simulink model "sim_model"  (R2015b)
settings: Solver=FixedStepDiscrete  SolverMode=SingleTasking  StartTime=0.0  StopTime=sim_len  FixedStep=1  RelTol=1e-3
undefined symbols (not defined in the file): A, B, C, ir_matrix, modulator_reg_1_address, modulator_reg_1_default, modulator_reg_1_num_bits, N_sub
libraries: xbsIndex_r4 x3875
(part 4 of 193)

== system sim_model/channelizer/poly_phase_filter1/filter_pipeline_89_taps3/8_taps ==
  delay_line_in : Inport
  result_in : Inport  Port=2
  reset_in : Inport  Port=3
  enable_in : Inport  Port=4
  one_tab_1 : Subsystem  mask{impulse_response_matrix=impulse_response_matrix(2,:), N_sub=N_sub}
      mask prompts: impulse_response_matrix "Tab IR"
  one_tab_2 : Subsystem  mask{impulse_response_matrix=impulse_response_matrix(4,:), N_sub=N_sub}
      mask prompts: impulse_response_matrix "Tab IR"
  one_tab_3 : Subsystem  mask{impulse_response_matrix=impulse_response_matrix(3,:), N_sub=N_sub}
      mask prompts: impulse_response_matrix "Tab IR"
  one_tab_4 : Subsystem  mask{impulse_response_matrix=impulse_response_matrix(6,:), N_sub=N_sub}
      mask prompts: impulse_response_matrix "Tab IR"
  one_tab_5 : Subsystem  mask{impulse_response_matrix=impulse_response_matrix(5,:), N_sub=N_sub}
      mask prompts: impulse_response_matrix "Tab IR"
  one_tab_6 : Subsystem  mask{impulse_response_matrix=impulse_response_matrix(8,:), N_sub=N_sub}
      mask prompts: impulse_response_matrix "Tab IR"
  one_tab_7 : Subsystem  mask{impulse_response_matrix=impulse_response_matrix(7,:), N_sub=N_sub}
      mask prompts: impulse_response_matrix "Tab IR"
  one_tab_8 : Subsystem  mask{impulse_response_matrix=impulse_response_matrix(1,:), N_sub=N_sub}
      mask prompts: impulse_response_matrix "Tab IR"
  delay_line_out : Outport
  result_out : Outport  Port=2
  reset_out : Outport  Port=3
  enable_out : Outport  Port=4
  wires:
  one_tab_6/1(delay_line_out) -> delay_line_out/1
  one_tab_6/2(result_out) -> result_out/1
  one_tab_6/3(reset_out) -> reset_out/1
  result_in/1 -> one_tab_8/2(result_in)
  delay_line_in/1 -> one_tab_8/1(delay_line_in)
  reset_in/1 -> one_tab_8/3(reset_in)
  enable_in/1 -> one_tab_8/4(enable_in)
  one_tab_6/4(enable_out) -> enable_out/1
  one_tab_8/1(delay_line_out) -> one_tab_1/1(delay_line_in)
  one_tab_8/2(result_out) -> one_tab_1/2(result_in)
  one_tab_8/3(reset_out) -> one_tab_1/3(reset_in)
  one_tab_8/4(enable_out) -> one_tab_1/4(enable_in)
  one_tab_3/1(delay_line_out) -> one_tab_2/1(delay_line_in)
  one_tab_3/2(result_out) -> one_tab_2/2(result_in)
  one_tab_3/3(reset_out) -> one_tab_2/3(reset_in)
  one_tab_3/4(enable_out) -> one_tab_2/4(enable_in)
  one_tab_1/1(delay_line_out) -> one_tab_3/1(delay_line_in)
  one_tab_1/2(result_out) -> one_tab_3/2(result_in)
  one_tab_1/3(reset_out) -> one_tab_3/3(reset_in)
  one_tab_1/4(enable_out) -> one_tab_3/4(enable_in)
  one_tab_5/1(delay_line_out) -> one_tab_4/1(delay_line_in)
  one_tab_5/2(result_out) -> one_tab_4/2(result_in)
  one_tab_5/3(reset_out) -> one_tab_4/3(reset_in)
  one_tab_5/4(enable_out) -> one_tab_4/4(enable_in)
  one_tab_2/1(delay_line_out) -> one_tab_5/1(delay_line_in)
  one_tab_2/2(result_out) -> one_tab_5/2(result_in)
  one_tab_2/3(reset_out) -> one_tab_5/3(reset_in)
  one_tab_2/4(enable_out) -> one_tab_5/4(enable_in)
  one_tab_7/1(delay_line_out) -> one_tab_6/1(delay_line_in)
  one_tab_7/2(result_out) -> one_tab_6/2(result_in)
  one_tab_7/3(reset_out) -> one_tab_6/3(reset_in)
  one_tab_7/4(enable_out) -> one_tab_6/4(enable_in)
  one_tab_4/1(delay_line_out) -> one_tab_7/1(delay_line_in)
  one_tab_4/2(result_out) -> one_tab_7/2(result_in)
  one_tab_4/3(reset_out) -> one_tab_7/3(reset_in)
  one_tab_4/4(enable_out) -> one_tab_7/4(enable_in)

== system sim_model/channelizer/poly_phase_filter1/filter_pipeline_89_taps3/8_taps1 ==
  delay_line_in : Inport
  result_in : Inport  Port=2
  reset_in : Inport  Port=3
  enable_in : Inport  Port=4
  one_tab_1 : Subsystem  mask{impulse_response_matrix=impulse_response_matrix(2,:), N_sub=N_sub}
      mask prompts: impulse_response_matrix "Tab IR"
  one_tab_2 : Subsystem  mask{impulse_response_matrix=impulse_response_matrix(4,:), N_sub=N_sub}
      mask prompts: impulse_response_matrix "Tab IR"
  one_tab_3 : Subsystem  mask{impulse_response_matrix=impulse_response_matrix(3,:), N_sub=N_sub}
      mask prompts: impulse_response_matrix "Tab IR"
  one_tab_4 : Subsystem  mask{impulse_response_matrix=impulse_response_matrix(6,:), N_sub=N_sub}
      mask prompts: impulse_response_matrix "Tab IR"
  one_tab_5 : Subsystem  mask{impulse_response_matrix=impulse_response_matrix(5,:), N_sub=N_sub}
      mask prompts: impulse_response_matrix "Tab IR"
  one_tab_6 : Subsystem  mask{impulse_response_matrix=impulse_response_matrix(8,:), N_sub=N_sub}
      mask prompts: impulse_response_matrix "Tab IR"
  one_tab_7 : Subsystem  mask{impulse_response_matrix=impulse_response_matrix(7,:), N_sub=N_sub}
      mask prompts: impulse_response_matrix "Tab IR"
  one_tab_8 : Subsystem  mask{impulse_response_matrix=impulse_response_matrix(1,:), N_sub=N_sub}
      mask prompts: impulse_response_matrix "Tab IR"
  delay_line_out : Outport
  result_out : Outport  Port=2
  reset_out : Outport  Port=3
  enable_out : Outport  Port=4
  wires:
  one_tab_6/1(delay_line_out) -> delay_line_out/1
  one_tab_6/2(result_out) -> result_out/1
  one_tab_6/3(reset_out) -> reset_out/1
  result_in/1 -> one_tab_8/2(result_in)
  delay_line_in/1 -> one_tab_8/1(delay_line_in)
  reset_in/1 -> one_tab_8/3(reset_in)
  enable_in/1 -> one_tab_8/4(enable_in)
  one_tab_6/4(enable_out) -> enable_out/1
  one_tab_8/1(delay_line_out) -> one_tab_1/1(delay_line_in)
  one_tab_8/2(result_out) -> one_tab_1/2(result_in)
  one_tab_8/3(reset_out) -> one_tab_1/3(reset_in)
  one_tab_8/4(enable_out) -> one_tab_1/4(enable_in)
  one_tab_3/1(delay_line_out) -> one_tab_2/1(delay_line_in)
  one_tab_3/2(result_out) -> one_tab_2/2(result_in)
  one_tab_3/3(reset_out) -> one_tab_2/3(reset_in)
  one_tab_3/4(enable_out) -> one_tab_2/4(enable_in)
  one_tab_1/1(delay_line_out) -> one_tab_3/1(delay_line_in)
  one_tab_1/2(result_out) -> one_tab_3/2(result_in)
  one_tab_1/3(reset_out) -> one_tab_3/3(reset_in)
  one_tab_1/4(enable_out) -> one_tab_3/4(enable_in)
  one_tab_5/1(delay_line_out) -> one_tab_4/1(delay_line_in)
  one_tab_5/2(result_out) -> one_tab_4/2(result_in)
  one_tab_5/3(reset_out) -> one_tab_4/3(reset_in)
  one_tab_5/4(enable_out) -> one_tab_4/4(enable_in)
  one_tab_2/1(delay_line_out) -> one_tab_5/1(delay_line_in)
  one_tab_2/2(result_out) -> one_tab_5/2(result_in)
  one_tab_2/3(reset_out) -> one_tab_5/3(reset_in)
  one_tab_2/4(enable_out) -> one_tab_5/4(enable_in)
  one_tab_7/1(delay_line_out) -> one_tab_6/1(delay_line_in)
  one_tab_7/2(result_out) -> one_tab_6/2(result_in)
  one_tab_7/3(reset_out) -> one_tab_6/3(reset_in)
  one_tab_7/4(enable_out) -> one_tab_6/4(enable_in)
  one_tab_4/1(delay_line_out) -> one_tab_7/1(delay_line_in)
  one_tab_4/2(result_out) -> one_tab_7/2(result_in)
  one_tab_4/3(reset_out) -> one_tab_7/3(reset_in)
  one_tab_4/4(enable_out) -> one_tab_7/4(enable_in)

== system sim_model/channelizer/poly_phase_filter1/filter_pipeline_89_taps3/8_taps10 ==
  delay_line_in : Inport
  result_in : Inport  Port=2
  reset_in : Inport  Port=3
  enable_in : Inport  Port=4
  one_tab_1 : Subsystem  mask{impulse_response_matrix=impulse_response_matrix(2,:), N_sub=N_sub}
      mask prompts: impulse_response_matrix "Tab IR"
  one_tab_2 : Subsystem  mask{impulse_response_matrix=impulse_response_matrix(4,:), N_sub=N_sub}
      mask prompts: impulse_response_matrix "Tab IR"
  one_tab_3 : Subsystem  mask{impulse_response_matrix=impulse_response_matrix(3,:), N_sub=N_sub}
      mask prompts: impulse_response_matrix "Tab IR"
  one_tab_4 : Subsystem  mask{impulse_response_matrix=impulse_response_matrix(6,:), N_sub=N_sub}
      mask prompts: impulse_response_matrix "Tab IR"
  one_tab_5 : Subsystem  mask{impulse_response_matrix=impulse_response_matrix(5,:), N_sub=N_sub}
      mask prompts: impulse_response_matrix "Tab IR"
  one_tab_6 : Subsystem  mask{impulse_response_matrix=impulse_response_matrix(8,:), N_sub=N_sub}
      mask prompts: impulse_response_matrix "Tab IR"
  one_tab_7 : Subsystem  mask{impulse_response_matrix=impulse_response_matrix(7,:), N_sub=N_sub}
      mask prompts: impulse_response_matrix "Tab IR"
  one_tab_8 : Subsystem  mask{impulse_response_matrix=impulse_response_matrix(1,:), N_sub=N_sub}
      mask prompts: impulse_response_matrix "Tab IR"
  delay_line_out : Outport
  result_out : Outport  Port=2
  reset_out : Outport  Port=3
  enable_out : Outport  Port=4
  wires:
  one_tab_6/1(delay_line_out) -> delay_line_out/1
  one_tab_6/2(result_out) -> result_out/1
  one_tab_6/3(reset_out) -> reset_out/1
  result_in/1 -> one_tab_8/2(result_in)
  delay_line_in/1 -> one_tab_8/1(delay_line_in)
  reset_in/1 -> one_tab_8/3(reset_in)
  enable_in/1 -> one_tab_8/4(enable_in)
  one_tab_6/4(enable_out) -> enable_out/1
  one_tab_8/1(delay_line_out) -> one_tab_1/1(delay_line_in)
  one_tab_8/2(result_out) -> one_tab_1/2(result_in)
  one_tab_8/3(reset_out) -> one_tab_1/3(reset_in)
  one_tab_8/4(enable_out) -> one_tab_1/4(enable_in)
  one_tab_3/1(delay_line_out) -> one_tab_2/1(delay_line_in)
  one_tab_3/2(result_out) -> one_tab_2/2(result_in)
  one_tab_3/3(reset_out) -> one_tab_2/3(reset_in)
  one_tab_3/4(enable_out) -> one_tab_2/4(enable_in)
  one_tab_1/1(delay_line_out) -> one_tab_3/1(delay_line_in)
  one_tab_1/2(result_out) -> one_tab_3/2(result_in)
  one_tab_1/3(reset_out) -> one_tab_3/3(reset_in)
  one_tab_1/4(enable_out) -> one_tab_3/4(enable_in)
  one_tab_5/1(delay_line_out) -> one_tab_4/1(delay_line_in)
  one_tab_5/2(result_out) -> one_tab_4/2(result_in)
  one_tab_5/3(reset_out) -> one_tab_4/3(reset_in)
  one_tab_5/4(enable_out) -> one_tab_4/4(enable_in)
  one_tab_2/1(delay_line_out) -> one_tab_5/1(delay_line_in)
  one_tab_2/2(result_out) -> one_tab_5/2(result_in)
  one_tab_2/3(reset_out) -> one_tab_5/3(reset_in)
  one_tab_2/4(enable_out) -> one_tab_5/4(enable_in)
  one_tab_7/1(delay_line_out) -> one_tab_6/1(delay_line_in)
  one_tab_7/2(result_out) -> one_tab_6/2(result_in)
  one_tab_7/3(reset_out) -> one_tab_6/3(reset_in)
  one_tab_7/4(enable_out) -> one_tab_6/4(enable_in)
  one_tab_4/1(delay_line_out) -> one_tab_7/1(delay_line_in)
  one_tab_4/2(result_out) -> one_tab_7/2(result_in)
  one_tab_4/3(reset_out) -> one_tab_7/3(reset_in)
  one_tab_4/4(enable_out) -> one_tab_7/4(enable_in)

== system sim_model/channelizer/poly_phase_filter1/filter_pipeline_89_taps3/8_taps2 ==
  delay_line_in : Inport
  result_in : Inport  Port=2
  reset_in : Inport  Port=3
  enable_in : Inport  Port=4
  one_tab_1 : Subsystem  mask{impulse_response_matrix=impulse_response_matrix(2,:), N_sub=N_sub}
      mask prompts: impulse_response_matrix "Tab IR"
  one_tab_2 : Subsystem  mask{impulse_response_matrix=impulse_response_matrix(4,:), N_sub=N_sub}
      mask prompts: impulse_response_matrix "Tab IR"
  one_tab_3 : Subsystem  mask{impulse_response_matrix=impulse_response_matrix(3,:), N_sub=N_sub}
      mask prompts: impulse_response_matrix "Tab IR"
  one_tab_4 : Subsystem  mask{impulse_response_matrix=impulse_response_matrix(6,:), N_sub=N_sub}
      mask prompts: impulse_response_matrix "Tab IR"
  one_tab_5 : Subsystem  mask{impulse_response_matrix=impulse_response_matrix(5,:), N_sub=N_sub}
      mask prompts: impulse_response_matrix "Tab IR"
  one_tab_6 : Subsystem  mask{impulse_response_matrix=impulse_response_matrix(8,:), N_sub=N_sub}
      mask prompts: impulse_response_matrix "Tab IR"
  one_tab_7 : Subsystem  mask{impulse_response_matrix=impulse_response_matrix(7,:), N_sub=N_sub}
      mask prompts: impulse_response_matrix "Tab IR"
  one_tab_8 : Subsystem  mask{impulse_response_matrix=impulse_response_matrix(1,:), N_sub=N_sub}
      mask prompts: impulse_response_matrix "Tab IR"
  delay_line_out : Outport
  result_out : Outport  Port=2
  reset_out : Outport  Port=3
  enable_out : Outport  Port=4
  wires:
  one_tab_6/1(delay_line_out) -> delay_line_out/1
  one_tab_6/2(result_out) -> result_out/1
  one_tab_6/3(reset_out) -> reset_out/1
  result_in/1 -> one_tab_8/2(result_in)
  delay_line_in/1 -> one_tab_8/1(delay_line_in)
  reset_in/1 -> one_tab_8/3(reset_in)
  enable_in/1 -> one_tab_8/4(enable_in)
  one_tab_6/4(enable_out) -> enable_out/1
  one_tab_8/1(delay_line_out) -> one_tab_1/1(delay_line_in)
  one_tab_8/2(result_out) -> one_tab_1/2(result_in)
  one_tab_8/3(reset_out) -> one_tab_1/3(reset_in)
  one_tab_8/4(enable_out) -> one_tab_1/4(enable_in)
  one_tab_3/1(delay_line_out) -> one_tab_2/1(delay_line_in)
  one_tab_3/2(result_out) -> one_tab_2/2(result_in)
  one_tab_3/3(reset_out) -> one_tab_2/3(reset_in)
  one_tab_3/4(enable_out) -> one_tab_2/4(enable_in)
  one_tab_1/1(delay_line_out) -> one_tab_3/1(delay_line_in)
  one_tab_1/2(result_out) -> one_tab_3/2(result_in)
  one_tab_1/3(reset_out) -> one_tab_3/3(reset_in)
  one_tab_1/4(enable_out) -> one_tab_3/4(enable_in)
  one_tab_5/1(delay_line_out) -> one_tab_4/1(delay_line_in)
  one_tab_5/2(result_out) -> one_tab_4/2(result_in)
  one_tab_5/3(reset_out) -> one_tab_4/3(reset_in)
  one_tab_5/4(enable_out) -> one_tab_4/4(enable_in)
  one_tab_2/1(delay_line_out) -> one_tab_5/1(delay_line_in)
  one_tab_2/2(result_out) -> one_tab_5/2(result_in)
  one_tab_2/3(reset_out) -> one_tab_5/3(reset_in)
  one_tab_2/4(enable_out) -> one_tab_5/4(enable_in)
  one_tab_7/1(delay_line_out) -> one_tab_6/1(delay_line_in)
  one_tab_7/2(result_out) -> one_tab_6/2(result_in)
  one_tab_7/3(reset_out) -> one_tab_6/3(reset_in)
  one_tab_7/4(enable_out) -> one_tab_6/4(enable_in)
  one_tab_4/1(delay_line_out) -> one_tab_7/1(delay_line_in)
  one_tab_4/2(result_out) -> one_tab_7/2(result_in)
  one_tab_4/3(reset_out) -> one_tab_7/3(reset_in)
  one_tab_4/4(enable_out) -> one_tab_7/4(enable_in)

== system sim_model/channelizer/poly_phase_filter1/filter_pipeline_89_taps3/8_taps3 ==
  delay_line_in : Inport
  result_in : Inport  Port=2
  reset_in : Inport  Port=3
  enable_in : Inport  Port=4
  one_tab_1 : Subsystem  mask{impulse_response_matrix=impulse_response_matrix(2,:), N_sub=N_sub}
      mask prompts: impulse_response_matrix "Tab IR"
  one_tab_2 : Subsystem  mask{impulse_response_matrix=impulse_response_matrix(4,:), N_sub=N_sub}
      mask prompts: impulse_response_matrix "Tab IR"
  one_tab_3 : Subsystem  mask{impulse_response_matrix=impulse_response_matrix(3,:), N_sub=N_sub}
      mask prompts: impulse_response_matrix "Tab IR"
  one_tab_4 : Subsystem  mask{impulse_response_matrix=impulse_response_matrix(6,:), N_sub=N_sub}
      mask prompts: impulse_response_matrix "Tab IR"
  one_tab_5 : Subsystem  mask{impulse_response_matrix=impulse_response_matrix(5,:), N_sub=N_sub}
      mask prompts: impulse_response_matrix "Tab IR"
  one_tab_6 : Subsystem  mask{impulse_response_matrix=impulse_response_matrix(8,:), N_sub=N_sub}
      mask prompts: impulse_response_matrix "Tab IR"
  one_tab_7 : Subsystem  mask{impulse_response_matrix=impulse_response_matrix(7,:), N_sub=N_sub}
      mask prompts: impulse_response_matrix "Tab IR"
  one_tab_8 : Subsystem  mask{impulse_response_matrix=impulse_response_matrix(1,:), N_sub=N_sub}
      mask prompts: impulse_response_matrix "Tab IR"
  delay_line_out : Outport
  result_out : Outport  Port=2
  reset_out : Outport  Port=3
  enable_out : Outport  Port=4
  wires:
  one_tab_6/1(delay_line_out) -> delay_line_out/1
  one_tab_6/2(result_out) -> result_out/1
  one_tab_6/3(reset_out) -> reset_out/1
  result_in/1 -> one_tab_8/2(result_in)
  delay_line_in/1 -> one_tab_8/1(delay_line_in)
  reset_in/1 -> one_tab_8/3(reset_in)
  enable_in/1 -> one_tab_8/4(enable_in)
  one_tab_6/4(enable_out) -> enable_out/1
  one_tab_8/1(delay_line_out) -> one_tab_1/1(delay_line_in)
  one_tab_8/2(result_out) -> one_tab_1/2(result_in)
  one_tab_8/3(reset_out) -> one_tab_1/3(reset_in)
  one_tab_8/4(enable_out) -> one_tab_1/4(enable_in)
  one_tab_3/1(delay_line_out) -> one_tab_2/1(delay_line_in)
  one_tab_3/2(result_out) -> one_tab_2/2(result_in)
  one_tab_3/3(reset_out) -> one_tab_2/3(reset_in)
  one_tab_3/4(enable_out) -> one_tab_2/4(enable_in)
  one_tab_1/1(delay_line_out) -> one_tab_3/1(delay_line_in)
  one_tab_1/2(result_out) -> one_tab_3/2(result_in)
  one_tab_1/3(reset_out) -> one_tab_3/3(reset_in)
  one_tab_1/4(enable_out) -> one_tab_3/4(enable_in)
  one_tab_5/1(delay_line_out) -> one_tab_4/1(delay_line_in)
  one_tab_5/2(result_out) -> one_tab_4/2(result_in)
  one_tab_5/3(reset_out) -> one_tab_4/3(reset_in)
  one_tab_5/4(enable_out) -> one_tab_4/4(enable_in)
  one_tab_2/1(delay_line_out) -> one_tab_5/1(delay_line_in)
  one_tab_2/2(result_out) -> one_tab_5/2(result_in)
  one_tab_2/3(reset_out) -> one_tab_5/3(reset_in)
  one_tab_2/4(enable_out) -> one_tab_5/4(enable_in)
  one_tab_7/1(delay_line_out) -> one_tab_6/1(delay_line_in)
  one_tab_7/2(result_out) -> one_tab_6/2(result_in)
  one_tab_7/3(reset_out) -> one_tab_6/3(reset_in)
  one_tab_7/4(enable_out) -> one_tab_6/4(enable_in)
  one_tab_4/1(delay_line_out) -> one_tab_7/1(delay_line_in)
  one_tab_4/2(result_out) -> one_tab_7/2(result_in)
  one_tab_4/3(reset_out) -> one_tab_7/3(reset_in)
  one_tab_4/4(enable_out) -> one_tab_7/4(enable_in)

== system sim_model/channelizer/poly_phase_filter1/filter_pipeline_89_taps3/8_taps4 ==
  delay_line_in : Inport
  result_in : Inport  Port=2
  reset_in : Inport  Port=3
  enable_in : Inport  Port=4
  one_tab_1 : Subsystem  mask{impulse_response_matrix=impulse_response_matrix(2,:), N_sub=N_sub}
      mask prompts: impulse_response_matrix "Tab IR"
  one_tab_2 : Subsystem  mask{impulse_response_matrix=impulse_response_matrix(4,:), N_sub=N_sub}
      mask prompts: impulse_response_matrix "Tab IR"
  one_tab_3 : Subsystem  mask{impulse_response_matrix=impulse_response_matrix(3,:), N_sub=N_sub}
      mask prompts: impulse_response_matrix "Tab IR"
  one_tab_4 : Subsystem  mask{impulse_response_matrix=impulse_response_matrix(6,:), N_sub=N_sub}
      mask prompts: impulse_response_matrix "Tab IR"
  one_tab_5 : Subsystem  mask{impulse_response_matrix=impulse_response_matrix(5,:), N_sub=N_sub}
      mask prompts: impulse_response_matrix "Tab IR"
  one_tab_6 : Subsystem  mask{impulse_response_matrix=impulse_response_matrix(8,:), N_sub=N_sub}
      mask prompts: impulse_response_matrix "Tab IR"
  one_tab_7 : Subsystem  mask{impulse_response_matrix=impulse_response_matrix(7,:), N_sub=N_sub}
      mask prompts: impulse_response_matrix "Tab IR"
  one_tab_8 : Subsystem  mask{impulse_response_matrix=impulse_response_matrix(1,:), N_sub=N_sub}
      mask prompts: impulse_response_matrix "Tab IR"
  delay_line_out : Outport
  result_out : Outport  Port=2
  reset_out : Outport  Port=3
  enable_out : Outport  Port=4
  wires:
  one_tab_6/1(delay_line_out) -> delay_line_out/1
  one_tab_6/2(result_out) -> result_out/1
  one_tab_6/3(reset_out) -> reset_out/1
  result_in/1 -> one_tab_8/2(result_in)
  delay_line_in/1 -> one_tab_8/1(delay_line_in)
  reset_in/1 -> one_tab_8/3(reset_in)
  enable_in/1 -> one_tab_8/4(enable_in)
  one_tab_6/4(enable_out) -> enable_out/1
  one_tab_8/1(delay_line_out) -> one_tab_1/1(delay_line_in)
  one_tab_8/2(result_out) -> one_tab_1/2(result_in)
  one_tab_8/3(reset_out) -> one_tab_1/3(reset_in)
  one_tab_8/4(enable_out) -> one_tab_1/4(enable_in)
  one_tab_3/1(delay_line_out) -> one_tab_2/1(delay_line_in)
  one_tab_3/2(result_out) -> one_tab_2/2(result_in)
  one_tab_3/3(reset_out) -> one_tab_2/3(reset_in)
  one_tab_3/4(enable_out) -> one_tab_2/4(enable_in)
  one_tab_1/1(delay_line_out) -> one_tab_3/1(delay_line_in)
  one_tab_1/2(result_out) -> one_tab_3/2(result_in)
  one_tab_1/3(reset_out) -> one_tab_3/3(reset_in)
  one_tab_1/4(enable_out) -> one_tab_3/4(enable_in)
  one_tab_5/1(delay_line_out) -> one_tab_4/1(delay_line_in)
  one_tab_5/2(result_out) -> one_tab_4/2(result_in)
  one_tab_5/3(reset_out) -> one_tab_4/3(reset_in)
  one_tab_5/4(enable_out) -> one_tab_4/4(enable_in)
  one_tab_2/1(delay_line_out) -> one_tab_5/1(delay_line_in)
  one_tab_2/2(result_out) -> one_tab_5/2(result_in)
  one_tab_2/3(reset_out) -> one_tab_5/3(reset_in)
  one_tab_2/4(enable_out) -> one_tab_5/4(enable_in)
  one_tab_7/1(delay_line_out) -> one_tab_6/1(delay_line_in)
  one_tab_7/2(result_out) -> one_tab_6/2(result_in)
  one_tab_7/3(reset_out) -> one_tab_6/3(reset_in)
  one_tab_7/4(enable_out) -> one_tab_6/4(enable_in)
  one_tab_4/1(delay_line_out) -> one_tab_7/1(delay_line_in)
  one_tab_4/2(result_out) -> one_tab_7/2(result_in)
  one_tab_4/3(reset_out) -> one_tab_7/3(reset_in)
  one_tab_4/4(enable_out) -> one_tab_7/4(enable_in)

== system sim_model/channelizer/poly_phase_filter1/filter_pipeline_89_taps3/8_taps5 ==
  delay_line_in : Inport
  result_in : Inport  Port=2
  reset_in : Inport  Port=3
  enable_in : Inport  Port=4
  one_tab_1 : Subsystem  mask{impulse_response_matrix=impulse_response_matrix(2,:), N_sub=N_sub}
      mask prompts: impulse_response_matrix "Tab IR"
  one_tab_2 : Subsystem  mask{impulse_response_matrix=impulse_response_matrix(4,:), N_sub=N_sub}
      mask prompts: impulse_response_matrix "Tab IR"
  one_tab_3 : Subsystem  mask{impulse_response_matrix=impulse_response_matrix(3,:), N_sub=N_sub}
      mask prompts: impulse_response_matrix "Tab IR"
  one_tab_4 : Subsystem  mask{impulse_response_matrix=impulse_response_matrix(6,:), N_sub=N_sub}
      mask prompts: impulse_response_matrix "Tab IR"
  one_tab_5 : Subsystem  mask{impulse_response_matrix=impulse_response_matrix(5,:), N_sub=N_sub}
      mask prompts: impulse_response_matrix "Tab IR"
  one_tab_6 : Subsystem  mask{impulse_response_matrix=impulse_response_matrix(8,:), N_sub=N_sub}
      mask prompts: impulse_response_matrix "Tab IR"
  one_tab_7 : Subsystem  mask{impulse_response_matrix=impulse_response_matrix(7,:), N_sub=N_sub}
      mask prompts: impulse_response_matrix "Tab IR"
  one_tab_8 : Subsystem  mask{impulse_response_matrix=impulse_response_matrix(1,:), N_sub=N_sub}
      mask prompts: impulse_response_matrix "Tab IR"
  delay_line_out : Outport
  result_out : Outport  Port=2
  reset_out : Outport  Port=3
  enable_out : Outport  Port=4
  wires:
  one_tab_6/1(delay_line_out) -> delay_line_out/1
  one_tab_6/2(result_out) -> result_out/1
  one_tab_6/3(reset_out) -> reset_out/1
  result_in/1 -> one_tab_8/2(result_in)
  delay_line_in/1 -> one_tab_8/1(delay_line_in)
  reset_in/1 -> one_tab_8/3(reset_in)
  enable_in/1 -> one_tab_8/4(enable_in)
  one_tab_6/4(enable_out) -> enable_out/1
  one_tab_8/1(delay_line_out) -> one_tab_1/1(delay_line_in)
  one_tab_8/2(result_out) -> one_tab_1/2(result_in)
  one_tab_8/3(reset_out) -> one_tab_1/3(reset_in)
  one_tab_8/4(enable_out) -> one_tab_1/4(enable_in)
  one_tab_3/1(delay_line_out) -> one_tab_2/1(delay_line_in)
  one_tab_3/2(result_out) -> one_tab_2/2(result_in)
  one_tab_3/3(reset_out) -> one_tab_2/3(reset_in)
  one_tab_3/4(enable_out) -> one_tab_2/4(enable_in)
  one_tab_1/1(delay_line_out) -> one_tab_3/1(delay_line_in)
  one_tab_1/2(result_out) -> one_tab_3/2(result_in)
  one_tab_1/3(reset_out) -> one_tab_3/3(reset_in)
  one_tab_1/4(enable_out) -> one_tab_3/4(enable_in)
  one_tab_5/1(delay_line_out) -> one_tab_4/1(delay_line_in)
  one_tab_5/2(result_out) -> one_tab_4/2(result_in)
  one_tab_5/3(reset_out) -> one_tab_4/3(reset_in)
  one_tab_5/4(enable_out) -> one_tab_4/4(enable_in)
  one_tab_2/1(delay_line_out) -> one_tab_5/1(delay_line_in)
  one_tab_2/2(result_out) -> one_tab_5/2(result_in)
  one_tab_2/3(reset_out) -> one_tab_5/3(reset_in)
  one_tab_2/4(enable_out) -> one_tab_5/4(enable_in)
  one_tab_7/1(delay_line_out) -> one_tab_6/1(delay_line_in)
  one_tab_7/2(result_out) -> one_tab_6/2(result_in)
  one_tab_7/3(reset_out) -> one_tab_6/3(reset_in)
  one_tab_7/4(enable_out) -> one_tab_6/4(enable_in)
  one_tab_4/1(delay_line_out) -> one_tab_7/1(delay_line_in)
  one_tab_4/2(result_out) -> one_tab_7/2(result_in)
  one_tab_4/3(reset_out) -> one_tab_7/3(reset_in)
  one_tab_4/4(enable_out) -> one_tab_7/4(enable_in)

== system sim_model/channelizer/poly_phase_filter1/filter_pipeline_89_taps3/8_taps6 ==
  delay_line_in : Inport
  result_in : Inport  Port=2
  reset_in : Inport  Port=3
  enable_in : Inport  Port=4
  one_tab_1 : Subsystem  mask{impulse_response_matrix=impulse_response_matrix(2,:), N_sub=N_sub}
      mask prompts: impulse_response_matrix "Tab IR"
  one_tab_2 : Subsystem  mask{impulse_response_matrix=impulse_response_matrix(4,:), N_sub=N_sub}
      mask prompts: impulse_response_matrix "Tab IR"
  one_tab_3 : Subsystem  mask{impulse_response_matrix=impulse_response_matrix(3,:), N_sub=N_sub}
      mask prompts: impulse_response_matrix "Tab IR"
  one_tab_4 : Subsystem  mask{impulse_response_matrix=impulse_response_matrix(6,:), N_sub=N_sub}
      mask prompts: impulse_response_matrix "Tab IR"
  one_tab_5 : Subsystem  mask{impulse_response_matrix=impulse_response_matrix(5,:), N_sub=N_sub}
      mask prompts: impulse_response_matrix "Tab IR"
  one_tab_6 : Subsystem  mask{impulse_response_matrix=impulse_response_matrix(8,:), N_sub=N_sub}
      mask prompts: impulse_response_matrix "Tab IR"
  one_tab_7 : Subsystem  mask{impulse_response_matrix=impulse_response_matrix(7,:), N_sub=N_sub}
      mask prompts: impulse_response_matrix "Tab IR"
  one_tab_8 : Subsystem  mask{impulse_response_matrix=impulse_response_matrix(1,:), N_sub=N_sub}
      mask prompts: impulse_response_matrix "Tab IR"
  delay_line_out : Outport
  result_out : Outport  Port=2
  reset_out : Outport  Port=3
  enable_out : Outport  Port=4
  wires:
  one_tab_6/1(delay_line_out) -> delay_line_out/1
  one_tab_6/2(result_out) -> result_out/1
  one_tab_6/3(reset_out) -> reset_out/1
  result_in/1 -> one_tab_8/2(result_in)
  delay_line_in/1 -> one_tab_8/1(delay_line_in)
  reset_in/1 -> one_tab_8/3(reset_in)
  enable_in/1 -> one_tab_8/4(enable_in)
  one_tab_6/4(enable_out) -> enable_out/1
  one_tab_8/1(delay_line_out) -> one_tab_1/1(delay_line_in)
  one_tab_8/2(result_out) -> one_tab_1/2(result_in)
  one_tab_8/3(reset_out) -> one_tab_1/3(reset_in)
  one_tab_8/4(enable_out) -> one_tab_1/4(enable_in)
  one_tab_3/1(delay_line_out) -> one_tab_2/1(delay_line_in)
  one_tab_3/2(result_out) -> one_tab_2/2(result_in)
  one_tab_3/3(reset_out) -> one_tab_2/3(reset_in)
  one_tab_3/4(enable_out) -> one_tab_2/4(enable_in)
  one_tab_1/1(delay_line_out) -> one_tab_3/1(delay_line_in)
  one_tab_1/2(result_out) -> one_tab_3/2(result_in)
  one_tab_1/3(reset_out) -> one_tab_3/3(reset_in)
  one_tab_1/4(enable_out) -> one_tab_3/4(enable_in)
  one_tab_5/1(delay_line_out) -> one_tab_4/1(delay_line_in)
  one_tab_5/2(result_out) -> one_tab_4/2(result_in)
  one_tab_5/3(reset_out) -> one_tab_4/3(reset_in)
  one_tab_5/4(enable_out) -> one_tab_4/4(enable_in)
  one_tab_2/1(delay_line_out) -> one_tab_5/1(delay_line_in)
  one_tab_2/2(result_out) -> one_tab_5/2(result_in)
  one_tab_2/3(reset_out) -> one_tab_5/3(reset_in)
  one_tab_2/4(enable_out) -> one_tab_5/4(enable_in)
  one_tab_7/1(delay_line_out) -> one_tab_6/1(delay_line_in)
  one_tab_7/2(result_out) -> one_tab_6/2(result_in)
  one_tab_7/3(reset_out) -> one_tab_6/3(reset_in)
  one_tab_7/4(enable_out) -> one_tab_6/4(enable_in)
  one_tab_4/1(delay_line_out) -> one_tab_7/1(delay_line_in)
  one_tab_4/2(result_out) -> one_tab_7/2(result_in)
  one_tab_4/3(reset_out) -> one_tab_7/3(reset_in)
  one_tab_4/4(enable_out) -> one_tab_7/4(enable_in)

== system sim_model/channelizer/poly_phase_filter1/filter_pipeline_89_taps3/8_taps7 ==
  delay_line_in : Inport
  result_in : Inport  Port=2
  reset_in : Inport  Port=3
  enable_in : Inport  Port=4
  one_tab_1 : Subsystem  mask{impulse_response_matrix=impulse_response_matrix(2,:), N_sub=N_sub}
      mask prompts: impulse_response_matrix "Tab IR"
  one_tab_2 : Subsystem  mask{impulse_response_matrix=impulse_response_matrix(4,:), N_sub=N_sub}
      mask prompts: impulse_response_matrix "Tab IR"
  one_tab_3 : Subsystem  mask{impulse_response_matrix=impulse_response_matrix(3,:), N_sub=N_sub}
      mask prompts: impulse_response_matrix "Tab IR"
  one_tab_4 : Subsystem  mask{impulse_response_matrix=impulse_response_matrix(6,:), N_sub=N_sub}
      mask prompts: impulse_response_matrix "Tab IR"
  one_tab_5 : Subsystem  mask{impulse_response_matrix=impulse_response_matrix(5,:), N_sub=N_sub}
      mask prompts: impulse_response_matrix "Tab IR"
  one_tab_6 : Subsystem  mask{impulse_response_matrix=impulse_response_matrix(8,:), N_sub=N_sub}
      mask prompts: impulse_response_matrix "Tab IR"
  one_tab_7 : Subsystem  mask{impulse_response_matrix=impulse_response_matrix(7,:), N_sub=N_sub}
      mask prompts: impulse_response_matrix "Tab IR"
  one_tab_8 : Subsystem  mask{impulse_response_matrix=impulse_response_matrix(1,:), N_sub=N_sub}
      mask prompts: impulse_response_matrix "Tab IR"
  delay_line_out : Outport
  result_out : Outport  Port=2
  reset_out : Outport  Port=3
  enable_out : Outport  Port=4
  wires:
  one_tab_6/1(delay_line_out) -> delay_line_out/1
  one_tab_6/2(result_out) -> result_out/1
  one_tab_6/3(reset_out) -> reset_out/1
  result_in/1 -> one_tab_8/2(result_in)
  delay_line_in/1 -> one_tab_8/1(delay_line_in)
  reset_in/1 -> one_tab_8/3(reset_in)
  enable_in/1 -> one_tab_8/4(enable_in)
  one_tab_6/4(enable_out) -> enable_out/1
  one_tab_8/1(delay_line_out) -> one_tab_1/1(delay_line_in)
  one_tab_8/2(result_out) -> one_tab_1/2(result_in)
  one_tab_8/3(reset_out) -> one_tab_1/3(reset_in)
  one_tab_8/4(enable_out) -> one_tab_1/4(enable_in)
  one_tab_3/1(delay_line_out) -> one_tab_2/1(delay_line_in)
  one_tab_3/2(result_out) -> one_tab_2/2(result_in)
  one_tab_3/3(reset_out) -> one_tab_2/3(reset_in)
  one_tab_3/4(enable_out) -> one_tab_2/4(enable_in)
  one_tab_1/1(delay_line_out) -> one_tab_3/1(delay_line_in)
  one_tab_1/2(result_out) -> one_tab_3/2(result_in)
  one_tab_1/3(reset_out) -> one_tab_3/3(reset_in)
  one_tab_1/4(enable_out) -> one_tab_3/4(enable_in)
  one_tab_5/1(delay_line_out) -> one_tab_4/1(delay_line_in)
  one_tab_5/2(result_out) -> one_tab_4/2(result_in)
  one_tab_5/3(reset_out) -> one_tab_4/3(reset_in)
  one_tab_5/4(enable_out) -> one_tab_4/4(enable_in)
  one_tab_2/1(delay_line_out) -> one_tab_5/1(delay_line_in)
  one_tab_2/2(result_out) -> one_tab_5/2(result_in)
  one_tab_2/3(reset_out) -> one_tab_5/3(reset_in)
  one_tab_2/4(enable_out) -> one_tab_5/4(enable_in)
  one_tab_7/1(delay_line_out) -> one_tab_6/1(delay_line_in)
  one_tab_7/2(result_out) -> one_tab_6/2(result_in)
  one_tab_7/3(reset_out) -> one_tab_6/3(reset_in)
  one_tab_7/4(enable_out) -> one_tab_6/4(enable_in)
  one_tab_4/1(delay_line_out) -> one_tab_7/1(delay_line_in)
  one_tab_4/2(result_out) -> one_tab_7/2(result_in)
  one_tab_4/3(reset_out) -> one_tab_7/3(reset_in)
  one_tab_4/4(enable_out) -> one_tab_7/4(enable_in)

== system sim_model/channelizer/poly_phase_filter1/filter_pipeline_89_taps3/8_taps8 ==
  delay_line_in : Inport
  result_in : Inport  Port=2
  reset_in : Inport  Port=3
  enable_in : Inport  Port=4
  one_tab_1 : Subsystem  mask{impulse_response_matrix=impulse_response_matrix(2,:), N_sub=N_sub}
      mask prompts: impulse_response_matrix "Tab IR"
  one_tab_2 : Subsystem  mask{impulse_response_matrix=impulse_response_matrix(4,:), N_sub=N_sub}
      mask prompts: impulse_response_matrix "Tab IR"
  one_tab_3 : Subsystem  mask{impulse_response_matrix=impulse_response_matrix(3,:), N_sub=N_sub}
      mask prompts: impulse_response_matrix "Tab IR"
  one_tab_4 : Subsystem  mask{impulse_response_matrix=impulse_response_matrix(6,:), N_sub=N_sub}
      mask prompts: impulse_response_matrix "Tab IR"
  one_tab_5 : Subsystem  mask{impulse_response_matrix=impulse_response_matrix(5,:), N_sub=N_sub}
      mask prompts: impulse_response_matrix "Tab IR"
  one_tab_6 : Subsystem  mask{impulse_response_matrix=impulse_response_matrix(8,:), N_sub=N_sub}
      mask prompts: impulse_response_matrix "Tab IR"
  one_tab_7 : Subsystem  mask{impulse_response_matrix=impulse_response_matrix(7,:), N_sub=N_sub}
      mask prompts: impulse_response_matrix "Tab IR"
  one_tab_8 : Subsystem  mask{impulse_response_matrix=impulse_response_matrix(1,:), N_sub=N_sub}
      mask prompts: impulse_response_matrix "Tab IR"
  delay_line_out : Outport
  result_out : Outport  Port=2
  reset_out : Outport  Port=3
  enable_out : Outport  Port=4
  wires:
  one_tab_6/1(delay_line_out) -> delay_line_out/1
  one_tab_6/2(result_out) -> result_out/1
  one_tab_6/3(reset_out) -> reset_out/1
  result_in/1 -> one_tab_8/2(result_in)
  delay_line_in/1 -> one_tab_8/1(delay_line_in)
  reset_in/1 -> one_tab_8/3(reset_in)
  enable_in/1 -> one_tab_8/4(enable_in)
  one_tab_6/4(enable_out) -> enable_out/1
  one_tab_8/1(delay_line_out) -> one_tab_1/1(delay_line_in)
  one_tab_8/2(result_out) -> one_tab_1/2(result_in)
  one_tab_8/3(reset_out) -> one_tab_1/3(reset_in)
  one_tab_8/4(enable_out) -> one_tab_1/4(enable_in)
  one_tab_3/1(delay_line_out) -> one_tab_2/1(delay_line_in)
  one_tab_3/2(result_out) -> one_tab_2/2(result_in)
  one_tab_3/3(reset_out) -> one_tab_2/3(reset_in)
  one_tab_3/4(enable_out) -> one_tab_2/4(enable_in)
  one_tab_1/1(delay_line_out) -> one_tab_3/1(delay_line_in)
  one_tab_1/2(result_out) -> one_tab_3/2(result_in)
  one_tab_1/3(reset_out) -> one_tab_3/3(reset_in)
  one_tab_1/4(enable_out) -> one_tab_3/4(enable_in)
  one_tab_5/1(delay_line_out) -> one_tab_4/1(delay_line_in)
  one_tab_5/2(result_out) -> one_tab_4/2(result_in)
  one_tab_5/3(reset_out) -> one_tab_4/3(reset_in)
  one_tab_5/4(enable_out) -> one_tab_4/4(enable_in)
  one_tab_2/1(delay_line_out) -> one_tab_5/1(delay_line_in)
  one_tab_2/2(result_out) -> one_tab_5/2(result_in)
  one_tab_2/3(reset_out) -> one_tab_5/3(reset_in)
  one_tab_2/4(enable_out) -> one_tab_5/4(enable_in)
  one_tab_7/1(delay_line_out) -> one_tab_6/1(delay_line_in)
  one_tab_7/2(result_out) -> one_tab_6/2(result_in)
  one_tab_7/3(reset_out) -> one_tab_6/3(reset_in)
  one_tab_7/4(enable_out) -> one_tab_6/4(enable_in)
  one_tab_4/1(delay_line_out) -> one_tab_7/1(delay_line_in)
  one_tab_4/2(result_out) -> one_tab_7/2(result_in)
  one_tab_4/3(reset_out) -> one_tab_7/3(reset_in)
  one_tab_4/4(enable_out) -> one_tab_7/4(enable_in)

== system sim_model/channelizer/poly_phase_filter1/filter_pipeline_89_taps3/8_taps9 ==
  delay_line_in : Inport
  result_in : Inport  Port=2
  reset_in : Inport  Port=3
  enable_in : Inport  Port=4
  one_tab_1 : Subsystem  mask{impulse_response_matrix=impulse_response_matrix(2,:), N_sub=N_sub}
      mask prompts: impulse_response_matrix "Tab IR"
  one_tab_2 : Subsystem  mask{impulse_response_matrix=impulse_response_matrix(4,:), N_sub=N_sub}
      mask prompts: impulse_response_matrix "Tab IR"
  one_tab_3 : Subsystem  mask{impulse_response_matrix=impulse_response_matrix(3,:), N_sub=N_sub}
      mask prompts: impulse_response_matrix "Tab IR"
  one_tab_4 : Subsystem  mask{impulse_response_matrix=impulse_response_matrix(6,:), N_sub=N_sub}
      mask prompts: impulse_response_matrix "Tab IR"
  one_tab_5 : Subsystem  mask{impulse_response_matrix=impulse_response_matrix(5,:), N_sub=N_sub}
      mask prompts: impulse_response_matrix "Tab IR"
  one_tab_6 : Subsystem  mask{impulse_response_matrix=impulse_response_matrix(8,:), N_sub=N_sub}
      mask prompts: impulse_response_matrix "Tab IR"
  one_tab_7 : Subsystem  mask{impulse_response_matrix=impulse_response_matrix(7,:), N_sub=N_sub}
      mask prompts: impulse_response_matrix "Tab IR"
  one_tab_8 : Subsystem  mask{impulse_response_matrix=impulse_response_matrix(1,:), N_sub=N_sub}
      mask prompts: impulse_response_matrix "Tab IR"
  delay_line_out : Outport
  result_out : Outport  Port=2
  reset_out : Outport  Port=3
  enable_out : Outport  Port=4
  wires:
  one_tab_6/1(delay_line_out) -> delay_line_out/1
  one_tab_6/2(result_out) -> result_out/1
  one_tab_6/3(reset_out) -> reset_out/1
  result_in/1 -> one_tab_8/2(result_in)
  delay_line_in/1 -> one_tab_8/1(delay_line_in)
  reset_in/1 -> one_tab_8/3(reset_in)
  enable_in/1 -> one_tab_8/4(enable_in)
  one_tab_6/4(enable_out) -> enable_out/1
  one_tab_8/1(delay_line_out) -> one_tab_1/1(delay_line_in)
  one_tab_8/2(result_out) -> one_tab_1/2(result_in)
  one_tab_8/3(reset_out) -> one_tab_1/3(reset_in)
  one_tab_8/4(enable_out) -> one_tab_1/4(enable_in)
  one_tab_3/1(delay_line_out) -> one_tab_2/1(delay_line_in)
  one_tab_3/2(result_out) -> one_tab_2/2(result_in)
  one_tab_3/3(reset_out) -> one_tab_2/3(reset_in)
  one_tab_3/4(enable_out) -> one_tab_2/4(enable_in)
  one_tab_1/1(delay_line_out) -> one_tab_3/1(delay_line_in)
  one_tab_1/2(result_out) -> one_tab_3/2(result_in)
  one_tab_1/3(reset_out) -> one_tab_3/3(reset_in)
  one_tab_1/4(enable_out) -> one_tab_3/4(enable_in)
  one_tab_5/1(delay_line_out) -> one_tab_4/1(delay_line_in)
  one_tab_5/2(result_out) -> one_tab_4/2(result_in)
  one_tab_5/3(reset_out) -> one_tab_4/3(reset_in)
  one_tab_5/4(enable_out) -> one_tab_4/4(enable_in)
  one_tab_2/1(delay_line_out) -> one_tab_5/1(delay_line_in)
  one_tab_2/2(result_out) -> one_tab_5/2(result_in)
  one_tab_2/3(reset_out) -> one_tab_5/3(reset_in)
  one_tab_2/4(enable_out) -> one_tab_5/4(enable_in)
  one_tab_7/1(delay_line_out) -> one_tab_6/1(delay_line_in)
  one_tab_7/2(result_out) -> one_tab_6/2(result_in)
  one_tab_7/3(reset_out) -> one_tab_6/3(reset_in)
  one_tab_7/4(enable_out) -> one_tab_6/4(enable_in)
  one_tab_4/1(delay_line_out) -> one_tab_7/1(delay_line_in)
  one_tab_4/2(result_out) -> one_tab_7/2(result_in)
  one_tab_4/3(reset_out) -> one_tab_7/3(reset_in)
  one_tab_4/4(enable_out) -> one_tab_7/4(enable_in)
